simulink model "SF051A_SnsrOffsLrng"  (R2013b)
settings: Solver=FixedStepDiscrete  SolverMode=SingleTasking  StartTime=0.0  StopTime=1  FixedStep=0.002  RelTol=1e-3
values from neighbouring files (symbols this model uses):
  ARCHGLBPRM_10MILLISEC_SEC_F32 = DataDict.Constant    [SF051A_SnsrOffsLrng_DataDict.m]
  ARCHGLBPRM_2MILLISEC_SEC_F32 = DataDict.Constant    [SF051A_SnsrOffsLrng_DataDict.m]
  ARCHGLBPRM_2PI_ULS_F32 = DataDict.Constant    [SF051A_SnsrOffsLrng_DataDict.m]
  ARCHGLBPRM_FLOATZEROTHD_ULS_F32 = DataDict.Constant    [SF051A_SnsrOffsLrng_DataDict.m]
  ARCHGLBPRM_PIOVER180_ULS_F32 = DataDict.Constant    [SF051A_SnsrOffsLrng_DataDict.m]
  CNV100MICROSECTOSEC_SECPERCNT_F32 = DataDict.Constant    [SF051A_SnsrOffsLrng_DataDict.m]
  COVRAMTRXNIT_ULS_F32 = DataDict.Constant    [SF051A_SnsrOffsLrng_DataDict.m]
  HWAGHILIM_HWDEG_F32 = DataDict.Constant    [SF051A_SnsrOffsLrng_DataDict.m]
  HWAUTHYTHD_ULS_F32 = DataDict.Constant    [SF051A_SnsrOffsLrng_DataDict.m]
  HWTQLRNGSTSLRND_CNT_U08 = DataDict.Constant    [SF051A_SnsrOffsLrng_DataDict.m]
  HWTQLRNGSTSNEGOFFS_CNT_U08 = DataDict.Constant    [SF051A_SnsrOffsLrng_DataDict.m]
  HWTQLRNGSTSNOTLRND_CNT_U08 = DataDict.Constant    [SF051A_SnsrOffsLrng_DataDict.m]
  HWTQLRNGSTSPOSOFFS_CNT_U08 = DataDict.Constant    [SF051A_SnsrOffsLrng_DataDict.m]
  HWTQLRNGSTSZEROOFFS_CNT_U08 = DataDict.Constant    [SF051A_SnsrOffsLrng_DataDict.m]
  IDYMTRX_ULS_F32 = DataDict.Constant    [SF051A_SnsrOffsLrng_DataDict.m]
  IVS10MS_ULSPERSEC_F32 = DataDict.Constant    [SF051A_SnsrOffsLrng_DataDict.m]
  LRNGFILTICON_ULS_F32 = DataDict.Constant    [SF051A_SnsrOffsLrng_DataDict.m]
  ONE_ULS_F32 = DataDict.Constant    [SF051A_SnsrOffsLrng_DataDict.m]
  SnsrOffsLrnd = DataDict.NVM    [SF051A_SnsrOffsLrng_DataDict.m]
  SnsrOffsLrngFctEna = DataDict.Calibration    [SF051A_SnsrOffsLrng_DataDict.m]
  SnsrOffsLrngHwAgLrngDrvgDstThd = DataDict.Calibration    [SF051A_SnsrOffsLrng_DataDict.m]
  SnsrOffsLrngHwAgLrngEna = DataDict.Calibration    [SF051A_SnsrOffsLrng_DataDict.m]
  SnsrOffsLrngHwAgLrngHwVelThd = DataDict.Calibration    [SF051A_SnsrOffsLrng_DataDict.m]
  SnsrOffsLrngHwAgLrngSysTqThd = DataDict.Calibration    [SF051A_SnsrOffsLrng_DataDict.m]
  SnsrOffsLrngHwAgLrngSysTqThdMed = DataDict.Calibration    [SF051A_SnsrOffsLrng_DataDict.m]
  SnsrOffsLrngHwAgLrngSysTqThdTrustd = DataDict.Calibration    [SF051A_SnsrOffsLrng_DataDict.m]
  SnsrOffsLrngHwAgLrngSysTqThdWide = DataDict.Calibration    [SF051A_SnsrOffsLrng_DataDict.m]
  SnsrOffsLrngHwAgLrngTi = DataDict.Calibration    [SF051A_SnsrOffsLrng_DataDict.m]
  SnsrOffsLrngHwAgLrngVehSpdThd = DataDict.Calibration    [SF051A_SnsrOffsLrng_DataDict.m]
  SnsrOffsLrngHwAgLrngYawOffsDbnd = DataDict.Calibration    [SF051A_SnsrOffsLrng_DataDict.m]
  SnsrOffsLrngHwAgLrngYawRateThd = DataDict.Calibration    [SF051A_SnsrOffsLrng_DataDict.m]
  SnsrOffsLrngHwAgOffsLim = DataDict.Calibration    [SF051A_SnsrOffsLrng_DataDict.m]
  SnsrOffsLrngHwTqLrngEna = DataDict.Calibration    [SF051A_SnsrOffsLrng_DataDict.m]
  SnsrOffsLrngHwTqLrngEnaTiThd = DataDict.Calibration    [SF051A_SnsrOffsLrng_DataDict.m]
  SnsrOffsLrngHwTqLrngHwAgDbnd = DataDict.Calibration    [SF051A_SnsrOffsLrng_DataDict.m]
  SnsrOffsLrngHwTqLrngHwAgThd = DataDict.Calibration    [SF051A_SnsrOffsLrng_DataDict.m]
  SnsrOffsLrngHwTqLrngHwTqThd = DataDict.Calibration    [SF051A_SnsrOffsLrng_DataDict.m]
  SnsrOffsLrngHwTqLrngHwTqZeroOffsThd = DataDict.Calibration    [SF051A_SnsrOffsLrng_DataDict.m]
  SnsrOffsLrngHwTqLrngHwVelThd = DataDict.Calibration    [SF051A_SnsrOffsLrng_DataDict.m]
  SnsrOffsLrngHwTqLrngMeasTi = DataDict.Calibration    [SF051A_SnsrOffsLrng_DataDict.m]
  SnsrOffsLrngHwTqLrngMeasTiScar = DataDict.Calibration    [SF051A_SnsrOffsLrng_DataDict.m]
  SnsrOffsLrngHwTqLrngSampleImbThd1 = DataDict.Calibration    [SF051A_SnsrOffsLrng_DataDict.m]
  SnsrOffsLrngHwTqLrngSampleImbThd2 = DataDict.Calibration    [SF051A_SnsrOffsLrng_DataDict.m]
  SnsrOffsLrngHwTqLrngSampleThd1 = DataDict.Calibration    [SF051A_SnsrOffsLrng_DataDict.m]
  SnsrOffsLrngHwTqLrngSampleThd2 = DataDict.Calibration    [SF051A_SnsrOffsLrng_DataDict.m]
  SnsrOffsLrngHwTqLrngTiWghtCoeff = DataDict.Calibration    [SF051A_SnsrOffsLrng_DataDict.m]
  SnsrOffsLrngHwTqLrngVehSpdThd = DataDict.Calibration    [SF051A_SnsrOffsLrng_DataDict.m]
  SnsrOffsLrngHwTqOffsLim = DataDict.Calibration    [SF051A_SnsrOffsLrng_DataDict.m]
  SnsrOffsLrngSampleCntForHwTqLrngRst = DataDict.Calibration    [SF051A_SnsrOffsLrng_DataDict.m]
  SnsrOffsLrngTqInpDetnPwrEstimnThd = DataDict.Calibration    [SF051A_SnsrOffsLrng_DataDict.m]
  SnsrOffsLrngTqInpDetnSinGenrAmp = DataDict.Calibration    [SF051A_SnsrOffsLrng_DataDict.m]
  SnsrOffsLrngTqInpDetnSinGenrFrq = DataDict.Calibration    [SF051A_SnsrOffsLrng_DataDict.m]
  SnsrOffsLrngTqInpDetnStg1FilGain = DataDict.Calibration    [SF051A_SnsrOffsLrng_DataDict.m]
  SnsrOffsLrngTqInpDetnStg1WinSize = DataDict.Calibration    [SF051A_SnsrOffsLrng_DataDict.m]
  SnsrOffsLrngTqInpDetnStg2FilGainCen = DataDict.Calibration    [SF051A_SnsrOffsLrng_DataDict.m]
  SnsrOffsLrngTqInpDetnStg2FilGainDwn = DataDict.Calibration    [SF051A_SnsrOffsLrng_DataDict.m]
  SnsrOffsLrngTqInpDetnStg2FilGainUp = DataDict.Calibration    [SF051A_SnsrOffsLrng_DataDict.m]
  SnsrOffsLrngTqInpDetnStg2WinSize = DataDict.Calibration    [SF051A_SnsrOffsLrng_DataDict.m]
  SnsrOffsLrngYawLrngEna = DataDict.Calibration    [SF051A_SnsrOffsLrng_DataDict.m]
  SnsrOffsLrngYawLrngHwAgThd = DataDict.Calibration    [SF051A_SnsrOffsLrng_DataDict.m]
  SnsrOffsLrngYawLrngTi = DataDict.Calibration    [SF051A_SnsrOffsLrng_DataDict.m]
  SnsrOffsLrngYawLrngYawAThd = DataDict.Calibration    [SF051A_SnsrOffsLrng_DataDict.m]
  SnsrOffsLrngYawOffsFrshTiThd = DataDict.Calibration    [SF051A_SnsrOffsLrng_DataDict.m]
  SnsrOffsLrngYawRateOffsLim = DataDict.Calibration    [SF051A_SnsrOffsLrng_DataDict.m]
  SPDCNVN_MTRPERSECPERKPH_F32 = DataDict.Constant    [SF051A_SnsrOffsLrng_DataDict.m]
  SysGlbPrmSysTqRat = DataDict.ImprtdCal    [SF051A_SnsrOffsLrng_DataDict.m]
  TISTEP10MS_MINS_F32 = DataDict.Constant    [SF051A_SnsrOffsLrng_DataDict.m]
  TQINPDETNLOGGAIN_ULS_F32 = DataDict.Constant    [SF051A_SnsrOffsLrng_DataDict.m]
  YAWELPDTIHILIM_MINS_F32 = DataDict.Constant    [SF051A_SnsrOffsLrng_DataDict.m]
  YAWRATENOISE_VEHDEGPERSEC_F32 = DataDict.Constant    [SF051A_SnsrOffsLrng_DataDict.m]
  ZERO_ULS_F32 = DataDict.Constant    [SF051A_SnsrOffsLrng_DataDict.m]
  ZEROVECT_ULS_F32 = DataDict.Constant    [SF051A_SnsrOffsLrng_DataDict.m]
undefined symbols (not defined in the file or in its folder): NvmGetErrSts1
libraries: Fil x34, NxtrLim x20, FixdToFloat x17, FloatToFixd x16, simulink x12, NxtrAbslt x12, NxtrNvM x8, NxtrMath x3
(part 7 of 12)

== system SF051A_SnsrOffsLrng/SnsrOffsLrng/SnsrOffsLrngPer2/Enable_Function/YOC ==
  note: Every execution loop of Periodic 2, the yaw rate freshness timer increments.  Using a loop counter instead of client calls
      | because the elapsed time is "frozen" across ignition cycles.  The counter is reset to zero when learning occurs.
  note: When vehicle conditions are right and all bus signals are valid, begin or continue learning.
  YawRateLrngEna : Inport
  YawRateFild : Inport  RequirementInfo="{'linktype_rmi_doors' '0000babd (/E-STEER Core/SubSystem Specifications/Application Functions/SF051A Sensor Offset Learning)' '#SF051A_100' 'true' 'REQ:  SF051A_100' '' } %GIDa_4788fb8c_6bdd_419e_be01_c723b642e277"  Port=2
  YawA : Inport  RequirementInfo="{'linktype_rmi_doors' '0000babd (/E-STEER Core/SubSystem Specifications/Application Functions/SF051A Sensor Offset Learning)' '#SF051A_99' 'true' 'REQ:  SF051A_99' '' } %GIDa_1132fb7b_54bf_40b1_acf5_f9054bb6ad26"  Port=3
  VehSpd : Inport  RequirementInfo="{'linktype_rmi_doors' '0000babd (/E-STEER Core/SubSystem Specifications/Application Functions/SF051A Sensor Offset Learning)' '#SF051A_102' 'true' 'REQ:  SF051A_102' '' } %GIDa_5315707f_4311_4e1a_9598_78d874dd3bdb"  Port=4
  HwAg : Inport  RequirementInfo="{'linktype_rmi_doors' '0000babd (/E-STEER Core/SubSystem Specifications/Application Functions/SF051A Sensor Offset Learning)' '#SF051A_101' 'true' 'REQ:  SF051A_101' '' } %GIDa_72eb9de4_dd58_44cc_88ca_111522a15ca4"  Port=5
  Add : Sum
  Constant : Constant  RequirementInfo="{'linktype_rmi_doors' '0000babd (/E-STEER Core/SubSystem Specifications/Application Functions/SF051A Sensor Offset Learning)' '#SF051A_111' 'true' 'REQ:  SF051A_111' '' ; 'linktype_rmi_doors' '0000babd (/E-STEER Core/SubSystem Specifications/Application Functions/SF051A Sensor Offset Learning)' '#SF051A_242' 'true' 'REQ:  SF051A_242' '' } %GIDa_883fb207_2bdb_43f4_8fbf_3d3c8800e308"  Value=SnsrOffsLrngYawOffsFrshTiThd  OutDataTypeStr=single
  Constant1 : Constant  Value=TISTEP10MS_MINS_F32  OutDataTypeStr=single
  Data Store Read : DataStoreRead  DataStoreName=SnsrOffsLrnd  DataStoreElements=SnsrOffsLrnd.YawRateElpdTi
  Data Store Write : DataStoreWrite  DataStoreName=SnsrOffsLrnd  DataStoreElements=SnsrOffsLrnd.YawRateElpdTi
  Data Store Write1 : DataStoreWrite  RequirementInfo="{'linktype_rmi_doors' '0000babd (/E-STEER Core/SubSystem Specifications/Application Functions/SF051A Sensor Offset Learning)' '#SF051A_112' 'true' 'REQ:  SF051A_112' '' } %GIDa_1386d18f_d052_4548_b025_86f8f1b54bd3"  DataStoreName=VehYawRateOffsFrsh
  Do nothing : Subsystem  TreatAsAtomicUnit=on
  If : If  RequirementInfo="{'linktype_rmi_doors' '0000babd (/E-STEER Core/SubSystem Specifications/Application Functions/SF051A Sensor Offset Learning)' '#SF051A_95' 'true' 'REQ:  SF051A_95' '' } %GIDa_5a0d1c96_ac6c_4e69_b879_396e00cbc286"  NumInputs=2  IfExpression=u1 & u2
  Learn : Subsystem  RequirementInfo="{'linktype_rmi_doors' '0000babd (/E-STEER Core/SubSystem Specifications/Application Functions/SF051A Sensor Offset Learning)' '#SF051A_94' 'true' 'REQ:  SF051A_94' '' } %GIDa_548ddfb5_a741_4714_aec1_02ee3ee42dbb"  TreatAsAtomicUnit=on
  Learning Conditions : Subsystem  RequirementInfo="{'linktype_rmi_doors' '0000babd (/E-STEER Core/SubSystem Specifications/Application Functions/SF051A Sensor Offset Learning)' '#SF051A_97' 'true' 'REQ:  SF051A_97' '' ; 'linktype_rmi_doors' '0000babd (/E-STEER Core/SubSystem Specifications/Application Functions/SF051A Sensor Offset Learning)' '#SF051A_96' 'true' 'REQ:  SF051A_96' '' } %GIDa_890fa9a9_e67d_4d09_8fef_362b51c9d8ff"
  LimStat_f32 : NxtrLim/LimStat_f32  LoLim=ZERO_ULS_F32  HiLim=SnsrOffsLrngYawOffsFrshTiThd
      settings: AttributesFormatString=|
      | Low Limit: %<LoLim>
      | High Limit:%<HiLim>
  Relational Operator : RelationalOperator  RequirementInfo="{'linktype_rmi_doors' '0000babd (/E-STEER Core/SubSystem Specifications/Application Functions/SF051A Sensor Offset Learning)' '#SF051A_111' 'true' 'REQ:  SF051A_111' '' ; 'linktype_rmi_doors' '0000babd (/E-STEER Core/SubSystem Specifications/Application Functions/SF051A Sensor Offset Learning)' '#SF051A_242' 'true' 'REQ:  SF051A_242' '' } %GIDa_100189d6_4f90_49af_8752_2852919b8786"  Operator=<=  OutDataTypeStr=boolean
  Subsystem5 : Subsystem  Description=|  mask(Copyright Information){none=on}
      | Copyright info block.                                               
      |                                                                     
      | Place copyright information at the top of every subsystem in design.
      mask prompts: none "No parameters"
      mask help: Place copyright information at the top of every subsystem in design.
      mask Display:
      | NxtrConf = 'Nexteer Confidential';
      | 
      | sys = bdroot; %handle for the current model ("system")
      | first = get_param(sys,'Created');
      | first = first(end-3:end);  %year is last four digits
      | 
      | last = get_param(sys,'LastModifiedDate');
      | if isempty(last)
      |     last = datestr(now,'yyyy');
      | else
      |     last = last(end-3:end);
      | end
      | 
      | if strcmp(first,last)
      |     fprintf('%s -- Copyright %s Nexteer',NxtrConf,first)
      | else
      |     fprintf('%s -- %s%s- %s Nexteer',NxtrConf,char(169),first,last)
      | end
  wires:
  YawRateFild/1 -> Learning Conditions/4(YawRateFild), Learn/1(YawRate)
  Learning Conditions/1(LrngCdnVld) -> If/2
  YawRateLrngEna/1 -> If/1
  VehSpd/1 -> Learning Conditions/1(VehSpd)
  HwAg/1 -> Learning Conditions/2(HwAg)
  If/1 -> Learn/Action
  Constant/1 -> Relational Operator/2
  Data Store Read/1 -> Add/1
  Constant1/1 -> Add/2
  Add/1 -> LimStat_f32/1, Relational Operator/1  "ElpsdTi"
  LimStat_f32/1 -> Data Store Write/1
  YawA/1 -> Learning Conditions/3(YawA)
  If/2 -> Do nothing/Action
  Relational Operator/1 -> Data Store Write1/1

== system SF051A_SnsrOffsLrng/SnsrOffsLrng/SetHwTqOffs/Reset Learning/GetRefTmr100MicroSec32bit/CopyRight2 ==

== system SF051A_SnsrOffsLrng/SnsrOffsLrng/SnsrOffsLrngInit1/NVM Management/Data Invalid/Subsystem5 ==

== system SF051A_SnsrOffsLrng/SnsrOffsLrng/SnsrOffsLrngInit1/NVM Management/Data Valid/Subsystem5 ==

== system SF051A_SnsrOffsLrng/SnsrOffsLrng/SnsrOffsLrngInit1/NVM Management/Not Enabled/Subsystem5 ==

== system SF051A_SnsrOffsLrng/SnsrOffsLrng/SnsrOffsLrngPer1/EnableLearning/Default_TqInpDetn/Subsystem5 ==

== system SF051A_SnsrOffsLrng/SnsrOffsLrng/SnsrOffsLrngPer1/EnableLearning/EnablingConditions/CheckLastMeasHwPos ==
  HwAg : Inport
  Abslt_f32_f32 : NxtrAbslt/Abslt_f32_f32  SFunctionSpec=single y1 = Abslt_f32_f32(single u1)
      settings: AttributesFormatString=%<Name>
  Constant : Constant  Value=SnsrOffsLrngHwTqLrngHwAgDbnd
  Data Store Read : DataStoreRead  DataStoreName=SnsrOffsLrnd  DataStoreElements=SnsrOffsLrnd.HwTqLrngHwAgRef
  FalseOut_KeepRef : Subsystem  TreatAsAtomicUnit=on
  FixdToFloat_f32_s16 : FixdToFloat/FixdToFloat_f32_s16  Param1=4
  If : If  IfExpression=u1
  Merge : Merge
  Relational Operator : RelationalOperator  OutDataTypeStr=boolean
  Subsystem5 : Subsystem  Description=|  mask(Copyright Information){none=on}
      | Copyright info block.                                               
      |                                                                     
      | Place copyright information at the top of every subsystem in design.
      mask prompts: none "No parameters"
      mask help: Place copyright information at the top of every subsystem in design.
      mask Display:
      | NxtrConf = 'Nexteer Confidential';
      | 
      | sys = bdroot; %handle for the current model ("system")
      | first = get_param(sys,'Created');
      | first = first(end-3:end);  %year is last four digits
      | 
      | last = get_param(sys,'LastModifiedDate');
      | if isempty(last)
      |     last = datestr(now,'yyyy');
      | else
      |     last = last(end-3:end);
      | end
      | 
      | if strcmp(first,last)
      |     fprintf('%s -- Copyright %s Nexteer',NxtrConf,first)
      | else
      |     fprintf('%s -- %s%s- %s Nexteer',NxtrConf,char(169),first,last)
      | end
  Subtract : Sum  Inputs=+-
  TrueOut_ResetRef : Subsystem  TreatAsAtomicUnit=on
  HwAgMoved : Outport
  wires:
  Relational Operator/1 -> If/1
  Constant/1 -> Relational Operator/2
  Data Store Read/1 -> FixdToFloat_f32_s16/1
  HwAg/1 -> Subtract/1
  Subtract/1 -> Abslt_f32_f32/1
  Abslt_f32_f32/1 -> Relational Operator/1
  If/1 -> TrueOut_ResetRef/Action
  TrueOut_ResetRef/1(HwAgMoved) -> Merge/1
  FalseOut_KeepRef/1(HwAgMoved) -> Merge/2
  If/2 -> FalseOut_KeepRef/Action
  Merge/1 -> HwAgMoved/1
  FixdToFloat_f32_s16/1 -> Subtract/2

== system SF051A_SnsrOffsLrng/SnsrOffsLrng/SnsrOffsLrngPer1/EnableLearning/EnablingConditions/Subsystem5 ==

== system SF051A_SnsrOffsLrng/SnsrOffsLrng/SnsrOffsLrngPer1/EnableLearning/Eval_Time/GetTiSpan100MicroSec32bit ==
  note: Subtract original reference time
  note: seconds
  note: microseconds
  note: counts
  note: Wrap-to-zero
  note: 1 count = 100 uSec
  note: Get current system time
  note: GetTiSpan100MicroSec32bit
  note: Created Aug 18, 2015
      | Modified Oct 21, 2015
      | Modified Oct 30, 2015
      | Kevin Derry
  RefTmr : Inport
  CopyRight2 : Subsystem  Description=|  mask(Copyright Information){none=on}
      | Copyright info block.                                               
      |                                                                     
      | Place copyright information at the top of every subsystem in design.
      mask prompts: none "No parameters"
      mask help: Place copyright information at the top of every subsystem in design.
      mask Display:
      | NxtrConf = 'Nexteer Confidential';
      | 
      | sys = bdroot; %handle for the current model ("system")
      | first = get_param(sys,'Created');
      | if(isempty(first))
      |     first = datestr(now,'yyyy');
      | else
      |     first = first(end-3:end);  %year is last four digits
      | end
      | 
      | last = get_param(sys,'LastModifiedDate');
      | if isempty(last)
      |     last = datestr(now,'yyyy');
      | else
      |     last = last(end-3:end);
      | end
      | 
      | if strcmp(first,last)
      |     fprintf('%s -- Copyright %s Nexteer',NxtrConf,first)
      | else
      |     fprintf('%s -- %s%s- %s Nexteer',NxtrConf,char(169),first,last)
      | end
  Count per uSec : Constant  Value=0.01
  Data Store Read1 : DataStoreRead  DataStoreName=SimnTi
  Data Type Conversion2 : DataTypeConversion  OutDataTypeStr=uint32
  Divide1 : Product  Inputs=**
  Divide2 : Product  Inputs=*/
  If : If  NumInputs=2  IfExpression=u1 >= u2
  Max Counts : Constant  Value=2^32-1
  Merge : Merge
  No wrapping : Subsystem  TreatAsAtomicUnit=on
  Product2 : Product
  Product3 : Product
  Rounding : Rounding
  Subtract3 : Sum  Inputs=+-
  Wrapping : Subsystem  TreatAsAtomicUnit=on
  uSec per Sec : Constant  Value=1000000
  TiSpan : Outport
  wires:
  Wrapping/1(Out1) -> Merge/2
  No wrapping/1(Out1) -> Merge/1
  If/2 -> Wrapping/Action
  If/1 -> No wrapping/Action
  Product3/1 -> Subtract3/2
  Subtract3/1 -> Data Type Conversion2/1
  Rounding/1 -> Product3/1
  Divide2/1 -> Rounding/1
  Max Counts/1 -> Divide2/2, Product3/2
  Divide1/1 -> Divide2/1, Subtract3/1
  Product2/1 -> Divide1/1
  Data Store Read1/1 -> Product2/1
  Count per uSec/1 -> Divide1/2
  uSec per Sec/1 -> Product2/2
  Merge/1 -> TiSpan/1
  RefTmr/1 -> If/2, No wrapping/2(ref), Wrapping/2(ref)
  Data Type Conversion2/1 -> If/1, No wrapping/1(new), Wrapping/1(new)

== system SF051A_SnsrOffsLrng/SnsrOffsLrng/SnsrOffsLrngPer1/EnableLearning/Eval_Time/Subsystem5 ==

== system SF051A_SnsrOffsLrng/SnsrOffsLrng/SnsrOffsLrngPer1/EnableLearning/False_Reset/GetRefTmr100MicroSec32bit ==
  note: 1 count = 100 uSec
  note: seconds
  note: microseconds
  note: counts
  note: Wrap-to-zero
  note: GetRefTmr100MicroSec32bit
  note: Created Aug 18, 2015
      | Modified Oct 21, 2015
      | Modified Oct 30, 2015
      | Kevin Derry
  CopyRight2 : Subsystem  Description=|  mask(Copyright Information){none=on}
      | Copyright info block.                                               
      |                                                                     
      | Place copyright information at the top of every subsystem in design.
      mask prompts: none "No parameters"
      mask help: Place copyright information at the top of every subsystem in design.
      mask Display:
      | NxtrConf = 'Nexteer Confidential';
      | 
      | sys = bdroot; %handle for the current model ("system")
      | first = get_param(sys,'Created');
      | if(isempty(first))
      |     first = datestr(now,'yyyy');
      | else
      |     first = first(end-3:end);  %year is last four digits
      | end
      | 
      | last = get_param(sys,'LastModifiedDate');
      | if isempty(last)
      |     last = datestr(now,'yyyy');
      | else
      |     last = last(end-3:end);
      | end
      | 
      | if strcmp(first,last)
      |     fprintf('%s -- Copyright %s Nexteer',NxtrConf,first)
      | else
      |     fprintf('%s -- %s%s- %s Nexteer',NxtrConf,char(169),first,last)
      | end
  Count per uSec : Constant  Value=0.01
  Data Store Read1 : DataStoreRead  DataStoreName=SimnTi
  Data Type Conversion1 : DataTypeConversion  OutDataTypeStr=uint32
  Divide1 : Product  Inputs=**
  Divide2 : Product  Inputs=*/
  Max Counts : Constant  Value=2^32-1
  Product1 : Product
  Product2 : Product
  Rounding : Rounding
  Subtract1 : Sum  Inputs=+-
  uSec per Sec : Constant  Value=1000000
  RefTmr : Outport
  wires:
  Product2/1 -> Subtract1/2
  Subtract1/1 -> Data Type Conversion1/1
  Rounding/1 -> Product2/1
  Divide2/1 -> Rounding/1
  Max Counts/1 -> Divide2/2, Product2/2
  Divide1/1 -> Divide2/1, Subtract1/1
  Product1/1 -> Divide1/1
  Count per uSec/1 -> Divide1/2
  uSec per Sec/1 -> Product1/2
  Data Type Conversion1/1 -> RefTmr/1
  Data Store Read1/1 -> Product1/1

== system SF051A_SnsrOffsLrng/SnsrOffsLrng/SnsrOffsLrngPer1/EnableLearning/False_Reset/Subsystem5 ==

== system SF051A_SnsrOffsLrng/SnsrOffsLrng/SnsrOffsLrngPer1/EnableLearning/Filter_HwTq/Subsystem5 ==

== system SF051A_SnsrOffsLrng/SnsrOffsLrng/SnsrOffsLrngPer1/EnableLearning/Perform_TqInpDetn/Do nothing ==
  Action Port : ActionPort  ActionType=else
  Subsystem5 : Subsystem  Description=|  mask(Copyright Information){none=on}
      | Copyright info block.                                               
      |                                                                     
      | Place copyright information at the top of every subsystem in design.
      mask prompts: none "No parameters"
      mask help: Place copyright information at the top of every subsystem in design.
      mask Display:
      | NxtrConf = 'Nexteer Confidential';
      | 
      | sys = bdroot; %handle for the current model ("system")
      | first = get_param(sys,'Created');
      | first = first(end-3:end);  %year is last four digits
      | 
      | last = get_param(sys,'LastModifiedDate');
      | if isempty(last)
      |     last = datestr(now,'yyyy');
      | else
      |     last = last(end-3:end);
      | end
      | 
      | if strcmp(first,last)
      |     fprintf('%s -- Copyright %s Nexteer',NxtrConf,first)
      | else
      |     fprintf('%s -- %s%s- %s Nexteer',NxtrConf,char(169),first,last)
      | end

== system SF051A_SnsrOffsLrng/SnsrOffsLrng/SnsrOffsLrngPer1/EnableLearning/Perform_TqInpDetn/ElapsedTime ==
  Add : Sum
  Data Store Read : DataStoreRead  DataStoreName=TqInpDetnEnaTi
  Data Store Write : DataStoreWrite  DataStoreName=TqInpDetnEnaTi
  LimStat_f32 : NxtrLim/LimStat_f32  LoLim=ZERO_ULS_F32  HiLim=HWTQLRNGTMRHILIM_SEC_F32
      settings: AttributesFormatString=|
      | Low Limit: %<LoLim>
      | High Limit:%<HiLim>
  Subsystem5 : Subsystem  Description=|  mask(Copyright Information){none=on}
      | Copyright info block.                                               
      |                                                                     
      | Place copyright information at the top of every subsystem in design.
      mask prompts: none "No parameters"
      mask help: Place copyright information at the top of every subsystem in design.
      mask Display:
      | NxtrConf = 'Nexteer Confidential';
      | 
      | sys = bdroot; %handle for the current model ("system")
      | first = get_param(sys,'Created');
      | first = first(end-3:end);  %year is last four digits
      | 
      | last = get_param(sys,'LastModifiedDate');
      | if isempty(last)
      |     last = datestr(now,'yyyy');
      | else
      |     last = last(end-3:end);
      | end
      | 
      | if strcmp(first,last)
      |     fprintf('%s -- Copyright %s Nexteer',NxtrConf,first)
      | else
      |     fprintf('%s -- %s%s- %s Nexteer',NxtrConf,char(169),first,last)
      | end
  Ts : Constant  Value=ARCHGLBPRM_2MILLISEC_SEC_F32
  TiEnad : Outport
  wires:
  Ts/1 -> Add/1
  Data Store Read/1 -> Add/2
  Add/1 -> LimStat_f32/1
  LimStat_f32/1 -> TiEnad/1, Data Store Write/1

== system SF051A_SnsrOffsLrng/SnsrOffsLrng/SnsrOffsLrngPer1/EnableLearning/Perform_TqInpDetn/Enable_PreProcessing ==
  note: Enable_PreProcessing == true
  TiEnad : Inport
  HwTqFild : Inport  Port=2
  Constant : Constant  Value=SnsrOffsLrngTqInpDetnPwrEstimnThd
  Constant2 : Constant  Value=ARCHGLBPRM_2MILLISEC_SEC_F32
  Display : DataStoreWrite  DataStoreName=dSnsrOffsLrngTqInpPrsntRaw
  False_Hold : Subsystem  TreatAsAtomicUnit=on
  If : If  NumInputs=2  IfExpression=u1 & u2  ElseIfExpressions=u1 & ~u2
  Merge_Present : Merge  Inputs=3
  Merge_Validity : Merge  Inputs=3
  Preprocessing : Subsystem
  Product : Product
  Relational Operator : RelationalOperator  OutDataTypeStr=boolean
  Relational Operator1 : RelationalOperator  Operator=>  OutDataTypeStr=boolean
  Subsystem5 : Subsystem  Description=|  mask(Copyright Information){none=on}
      | Copyright info block.                                               
      |                                                                     
      | Place copyright information at the top of every subsystem in design.
      mask prompts: none "No parameters"
      mask help: Place copyright information at the top of every subsystem in design.
      mask Display:
      | NxtrConf = 'Nexteer Confidential';
      | 
      | sys = bdroot; %handle for the current model ("system")
      | first = get_param(sys,'Created');
      | first = first(end-3:end);  %year is last four digits
      | 
      | last = get_param(sys,'LastModifiedDate');
      | if isempty(last)
      |     last = datestr(now,'yyyy');
      | else
      |     last = last(end-3:end);
      | end
      | 
      | if strcmp(first,last)
      |     fprintf('%s -- Copyright %s Nexteer',NxtrConf,first)
      | else
      |     fprintf('%s -- %s%s- %s Nexteer',NxtrConf,char(169),first,last)
      | end
  True_False : Subsystem  TreatAsAtomicUnit=on
  True_True : Subsystem  TreatAsAtomicUnit=on
  TqInpPrsntVld : Outport  InitialOutput=0
  TqInpPrsnt : Outport  Port=2  InitialOutput=0
  wires:
  Preprocessing/2(HwTrqPreproc) -> Relational Operator1/1
  HwTqFild/1 -> Preprocessing/1(HwTqFild)
  Product/1 -> Relational Operator/2  "TqInpDetnBufTi"
  TiEnad/1 -> Relational Operator/1
  If/3 -> False_Hold/Action
  If/1 -> True_True/Action
  Relational Operator/1 -> If/1  "HwTqPreprocVld"
  Constant/1 -> Relational Operator1/2
  Relational Operator1/1 -> If/2, Display/1  "TqInpPrsntRaw"
  If/2 -> True_False/Action
  True_True/1(Vld) -> Merge_Validity/1
  True_False/1(Vld) -> Merge_Validity/2
  False_Hold/1(Vld) -> Merge_Validity/3
  Merge_Validity/1 -> TqInpPrsntVld/1
  True_True/2(Prsnt) -> Merge_Present/1
  True_False/2(Prsnt) -> Merge_Present/2
  False_Hold/2(Prsnt) -> Merge_Present/3
  Merge_Present/1 -> TqInpPrsnt/1
  Preprocessing/1(SampleCntrLim) -> Product/2
  Constant2/1 -> Product/1

== system SF051A_SnsrOffsLrng/SnsrOffsLrng/SnsrOffsLrngPer1/EnableLearning/Perform_TqInpDetn/SetStuffToZero ==
  Action Port : ActionPort  ActionType=then
  Constant : Constant  Value=ZERO_ULS_F32  OutDataTypeStr=single
      settings: AttributesFormatString=%<OutDataTypeStr>
  Constant1 : Constant  Value=0  OutDataTypeStr=uint16
      settings: AttributesFormatString=%<OutDataTypeStr>
  Constant2 : Constant  Value=0*(1:72)  OutDataTypeStr=single
      settings: AttributesFormatString=%<OutDataTypeStr>
  Constant3 : Constant  Value=true  OutDataTypeStr=boolean
      settings: AttributesFormatString=%<OutDataTypeStr>
  Constant4 : Constant  Value=0  OutDataTypeStr=uint8
      settings: AttributesFormatString=%<OutDataTypeStr>
  Data Store Write : DataStoreWrite  DataStoreName=TqInpDetnEnaTi
  Data Store Write1 : DataStoreWrite  DataStoreName=TqInpDetnHwTqFil  DataStoreElements=TqInpDetnHwTqFil.FilSt
  Data Store Write10 : DataStoreWrite  DataStoreName=TqInpDetnStg2UpFilSt2
  Data Store Write11 : DataStoreWrite  DataStoreName=TqInpDetnStg2UpFilSt1
  Data Store Write12 : DataStoreWrite  DataStoreName=TqInpDetnStg2CenFilSt1
  Data Store Write13 : DataStoreWrite  DataStoreName=TqInpDetnHwTqPreProc
  Data Store Write14 : DataStoreWrite  DataStoreName=TqInpDetnStg2DwnFilSt1
  Data Store Write15 : DataStoreWrite  DataStoreName=TqInpDetnStg2CenFilSt2
  Data Store Write2 : DataStoreWrite  DataStoreName=TqInpDetnPreProcEnaLoop
  Data Store Write4 : DataStoreWrite  DataStoreName=TqInpDetnSinGenrAg
  Data Store Write5 : DataStoreWrite  DataStoreName=TqInpDetnStg1Buf
  Data Store Write6 : DataStoreWrite  DataStoreName=TqInpDetnStg1Idx
  Data Store Write7 : DataStoreWrite  DataStoreName=TqInpDetnStg1FilSt2
  Data Store Write8 : DataStoreWrite  DataStoreName=TqInpDetnStg1FilSt1
  Data Store Write9 : DataStoreWrite  DataStoreName=TqInpDetnStg2DwnFilSt2
  StateVariable : DataStoreWrite  DataStoreName=HwTqLrngTqInpPrsnt
  Subsystem5 : Subsystem  Description=|  mask(Copyright Information){none=on}
      | Copyright info block.                                               
      |                                                                     
      | Place copyright information at the top of every subsystem in design.
      mask prompts: none "No parameters"
      mask help: Place copyright information at the top of every subsystem in design.
      mask Display:
      | NxtrConf = 'Nexteer Confidential';
      | 
      | sys = bdroot; %handle for the current model ("system")
      | first = get_param(sys,'Created');
      | first = first(end-3:end);  %year is last four digits
      | 
      | last = get_param(sys,'LastModifiedDate');
      | if isempty(last)
      |     last = datestr(now,'yyyy');
      | else
      |     last = last(end-3:end);
      | end
      | 
      | if strcmp(first,last)
      |     fprintf('%s -- Copyright %s Nexteer',NxtrConf,first)
      | else
      |     fprintf('%s -- %s%s- %s Nexteer',NxtrConf,char(169),first,last)
      | end
  wires:
  Constant1/1 -> Data Store Write2/1
  Constant/1 -> Data Store Write1/1, Data Store Write13/1, Data Store Write11/1, Data Store Write10/1, Data Store Write12/1, Data Store Write15/1, Data Store Write14/1, Data Store Write9/1, Data Store Write8/1, Data Store Write7/1, Data Store Write4/1, Data Store Write/1
  Constant2/1 -> Data Store Write5/1
  Constant3/1 -> StateVariable/1
  Constant4/1 -> Data Store Write6/1

== system SF051A_SnsrOffsLrng/SnsrOffsLrng/SnsrOffsLrngPer1/EnableLearning/Perform_TqInpDetn/Subsystem5 ==

== system SF051A_SnsrOffsLrng/SnsrOffsLrng/SnsrOffsLrngPer1/Learning/CalculateOnCenterTorqueDrift/Subsystem5 ==

== system SF051A_SnsrOffsLrng/SnsrOffsLrng/SnsrOffsLrngPer1/Learning/Counter/Increment_SampleCntNeg ==
  Action Port : ActionPort  ActionType=else
  " Constant" : Constant  OutDataTypeStr=uint16
      settings: AttributesFormatString=%<OutDataTypeStr>
  Add : Sum
  Data Store Read : DataStoreRead  DataStoreName=SnsrOffsLrnd  DataStoreElements=SnsrOffsLrnd.HwTqLrngSampleCntNeg
  Data Store Write : DataStoreWrite  DataStoreName=SnsrOffsLrnd  DataStoreElements=SnsrOffsLrnd.HwTqLrngSampleCntNeg
  Subsystem5 : Subsystem  Description=|  mask(Copyright Information){none=on}
      | Copyright info block.                                               
      |                                                                     
      | Place copyright information at the top of every subsystem in design.
      mask prompts: none "No parameters"
      mask help: Place copyright information at the top of every subsystem in design.
      mask Display:
      | NxtrConf = 'Nexteer Confidential';
      | 
      | sys = bdroot; %handle for the current model ("system")
      | first = get_param(sys,'Created');
      | first = first(end-3:end);  %year is last four digits
      | 
      | last = get_param(sys,'LastModifiedDate');
      | if isempty(last)
      |     last = datestr(now,'yyyy');
      | else
      |     last = last(end-3:end);
      | end
      | 
      | if strcmp(first,last)
      |     fprintf('%s -- Copyright %s Nexteer',NxtrConf,first)
      | else
      |     fprintf('%s -- %s%s- %s Nexteer',NxtrConf,char(169),first,last)
      | end
  Size : Outport
  wires:
  " Constant"/1 -> Add/1
  Add/1 -> Size/1, Data Store Write/1
  Data Store Read/1 -> Add/2

== system SF051A_SnsrOffsLrng/SnsrOffsLrng/SnsrOffsLrngPer1/Learning/Counter/Increment_SampleCntPos ==
  Action Port : ActionPort  ActionType=then
  "  Constant" : Constant  OutDataTypeStr=uint16
      settings: AttributesFormatString=%<OutDataTypeStr>
  Add : Sum
  Data Store Read : DataStoreRead  DataStoreName=SnsrOffsLrnd  DataStoreElements=SnsrOffsLrnd.HwTqLrngSampleCntPos
  Data Store Write : DataStoreWrite  DataStoreName=SnsrOffsLrnd  DataStoreElements=SnsrOffsLrnd.HwTqLrngSampleCntPos
  Subsystem5 : Subsystem  Description=|  mask(Copyright Information){none=on}
      | Copyright info block.                                               
      |                                                                     
      | Place copyright information at the top of every subsystem in design.
      mask prompts: none "No parameters"
      mask help: Place copyright information at the top of every subsystem in design.
      mask Display:
      | NxtrConf = 'Nexteer Confidential';
      | 
      | sys = bdroot; %handle for the current model ("system")
      | first = get_param(sys,'Created');
      | first = first(end-3:end);  %year is last four digits
      | 
      | last = get_param(sys,'LastModifiedDate');
      | if isempty(last)
      |     last = datestr(now,'yyyy');
      | else
      |     last = last(end-3:end);
      | end
      | 
      | if strcmp(first,last)
      |     fprintf('%s -- Copyright %s Nexteer',NxtrConf,first)
      | else
      |     fprintf('%s -- %s%s- %s Nexteer',NxtrConf,char(169),first,last)
      | end
  Size : Outport
  wires:
  "  Constant"/1 -> Add/1
  Add/1 -> Data Store Write/1, Size/1
  Data Store Read/1 -> Add/2

== system SF051A_SnsrOffsLrng/SnsrOffsLrng/SnsrOffsLrngPer1/Learning/Counter/Subsystem5 ==

== system SF051A_SnsrOffsLrng/SnsrOffsLrng/SnsrOffsLrngPer1/Learning/Do nothing/Subsystem5 ==

== system SF051A_SnsrOffsLrng/SnsrOffsLrng/SnsrOffsLrngPer1/Learning/ForgettingFactor/ResetHwTqLrng ==
  note: LPFs
  note: State Variables
  note: NVM
  Action Port : ActionPort  ActionType=then
  Constant1 : Constant  Value=ZERO_ULS_F32  OutDataTypeStr=single
      settings: AttributesFormatString=%<OutDataTypeStr>
  Constant10 : Constant  Value=true  OutDataTypeStr=boolean
      settings: AttributesFormatString=%<OutDataTypeStr>
  Constant3 : Constant  Value=HWAGHILIM_HWDEG_F32  OutDataTypeStr=single
      settings: AttributesFormatString=%<OutDataTypeStr>
  Constant4 : Constant  Value=IDYMTRX_ULS_F32  VectorParams1D=off  OutDataTypeStr=single
      settings: AttributesFormatString=%<OutDataTypeStr>, 3x3
  Constant5 : Constant  Value=0  OutDataTypeStr=uint16
      settings: AttributesFormatString=%<OutDataTypeStr>
  Constant7 : Constant  Value=ZEROVECT_ULS_F32  VectorParams1D=off  OutDataTypeStr=single
      settings: AttributesFormatString=%<OutDataTypeStr>, 3x1
  Constant8 : Constant  Value=COVRAMTRXNIT_ULS_F32  OutDataTypeStr=single
      settings: AttributesFormatString=%<OutDataTypeStr>
  Constant9 : Constant  Value=false  OutDataTypeStr=boolean
      settings: AttributesFormatString=%<OutDataTypeStr>
  Data Store Write1 : DataStoreWrite  DataStoreName=HwTqLrngEnaTmrRef
  Data Store Write10 : DataStoreWrite  DataStoreName=HwTqLrngTqInpPrsnt
  Data Store Write2 : DataStoreWrite  DataStoreName=HwTqLrngMeasTmrRef
  Data Store Write4 : DataStoreWrite  DataStoreName=HwAgMeasFil1  DataStoreElements=HwAgMeasFil1.FilSt
  Data Store Write5 : DataStoreWrite  DataStoreName=HwAgMeasFil2  DataStoreElements=HwAgMeasFil2.FilSt
  Data Store Write6 : DataStoreWrite  DataStoreName=HwTqMeasFil1  DataStoreElements=HwTqMeasFil1.FilSt
  Data Store Write7 : DataStoreWrite  DataStoreName=HwTqMeasFil2  DataStoreElements=HwTqMeasFil2.FilSt
  Data Store Write8 : DataStoreWrite  DataStoreName=HwTqLrngTqInpDetnEnaPrev
  Data Store Write9 : DataStoreWrite  DataStoreName=TqInpDetnHwTqFil  DataStoreElements=TqInpDetnHwTqFil.FilSt
  FloatToFixd_s16_f32 : FloatToFixd/FloatToFixd_s16_f32  Param1=4
  GetRefTmr100MicroSec32bit : Subsystem
  Product : Product
  Subsystem5 : Subsystem  Description=|  mask(Copyright Information){none=on}
      | Copyright info block.                                               
      |                                                                     
      | Place copyright information at the top of every subsystem in design.
      mask prompts: none "No parameters"
      mask help: Place copyright information at the top of every subsystem in design.
      mask Display:
      | NxtrConf = 'Nexteer Confidential';
      | 
      | sys = bdroot; %handle for the current model ("system")
      | first = get_param(sys,'Created');
      | first = first(end-3:end);  %year is last four digits
      | 
      | last = get_param(sys,'LastModifiedDate');
      | if isempty(last)
      |     last = datestr(now,'yyyy');
      | else
      |     last = last(end-3:end);
      | end
      | 
      | if strcmp(first,last)
      |     fprintf('%s -- Copyright %s Nexteer',NxtrConf,first)
      | else
      |     fprintf('%s -- %s%s- %s Nexteer',NxtrConf,char(169),first,last)
      | end
  Update NVM RAM : DataStoreWrite  DataStoreName=SnsrOffsLrnd  DataStoreElements=SnsrOffsLrnd.HwTqLrngSampleCntNeg#SnsrOffsLrnd.HwTqLrngSampleCntPos#SnsrOffsLrnd.HwTqLrngHwAgRef#SnsrOffsLrnd.HwTqLrngEstimnVect(:,:)#SnsrOffsLrnd.HwTqLrngCovariMtrx(:,:)
  wires:
  Constant1/1 -> Data Store Write9/1, Data Store Write7/1, Data Store Write6/1, Data Store Write5/1, Data Store Write4/1
  GetRefTmr100MicroSec32bit/1(RefTmr) -> Data Store Write2/1, Data Store Write1/1
  Constant3/1 -> FloatToFixd_s16_f32/1
  Constant5/1 -> Update NVM RAM/1, Update NVM RAM/2
  Constant4/1 -> Product/1
  Constant8/1 -> Product/2
  Product/1 -> Update NVM RAM/5
  Constant9/1 -> Data Store Write8/1
  Constant10/1 -> Data Store Write10/1
  FloatToFixd_s16_f32/1 -> Update NVM RAM/3
  Constant7/1 -> Update NVM RAM/4

== system SF051A_SnsrOffsLrng/SnsrOffsLrng/SnsrOffsLrngPer1/Learning/ForgettingFactor/Subsystem5 ==

== system SF051A_SnsrOffsLrng/SnsrOffsLrng/SnsrOffsLrngPer1/Learning/HwPos vs HwTrq Model/Subsystem5 ==

== system SF051A_SnsrOffsLrng/SnsrOffsLrng/SnsrOffsLrngPer1/Learning/Recursive Least Square Regression/Calculate Covariance Matrix ==
  note: 'SnsrOffsLrngHwTqLrngTiWghtCoeff' removed from here
  note: (X^T)*(X)
  note: X_k
  note: Mathworks
      | Reference
      | Frame
  note: 3x3
  note: 1x3
  note: 3x1
  note: 3x3
  note: 3x3
  note: 3x3
  note: 3x3
  note: CovMat_k = (I - KVect*XArry)*((CovMat_kPrev)/FF)
      |
      | Where:
      | I = Identity Matrix
      | CovMat_kPrev = Covariance Matrix result the previous iteration.
      | FF = Forgetting Factor (TiWghtCoeff, Time Weight Coefficient)
  XAry : Inport
  KVect : Inport  Port=2
  Data Store Read : DataStoreRead  DataStoreName=SnsrOffsLrnd  DataStoreElements=SnsrOffsLrnd.HwTqLrngCovariMtrx(:,:)
  Data Store Write : DataStoreWrite  RequirementInfo="{'linktype_rmi_doors' '0000babd (/E-STEER Core/SubSystem Specifications/Application Functions/SF051A Sensor Offset Learning)' '#SF051A_174' 'true' 'REQ: SF051A_174' '' ; 'linktype_rmi_doors' '0000babd (/E-STEER Core/SubSystem Specifications/Application Functions/SF051A Sensor Offset Learning)' '#SF051A_173' 'true' 'REQ:  SF051A_173' '' } %GIDa_53e9f122_ab02_4cc9_a40c_de49ec817421"  DataStoreName=SnsrOffsLrnd  DataStoreElements=SnsrOffsLrnd.HwTqLrngCovariMtrx(:,:)
  Identity Matrix : Constant  Value=IDYMTRX_ULS_F32  VectorParams1D=off  OutDataTypeStr=single
  Product : Product  Multiplication=Matrix(*)
  Product1 : Product  Multiplication=Matrix(*)
  Subsystem5 : Subsystem  Description=|  mask(Copyright Information){none=on}
      | Copyright info block.                                               
      |                                                                     
      | Place copyright information at the top of every subsystem in design.
      mask prompts: none "No parameters"
      mask help: Place copyright information at the top of every subsystem in design.
      mask Display:
      | NxtrConf = 'Nexteer Confidential';
      | 
      | sys = bdroot; %handle for the current model ("system")
      | first = get_param(sys,'Created');
      | first = first(end-3:end);  %year is last four digits
      | 
      | last = get_param(sys,'LastModifiedDate');
      | if isempty(last)
      |     last = datestr(now,'yyyy');
      | else
      |     last = last(end-3:end);
      | end
      | 
      | if strcmp(first,last)
      |     fprintf('%s -- Copyright %s Nexteer',NxtrConf,first)
      | else
      |     fprintf('%s -- %s%s- %s Nexteer',NxtrConf,char(169),first,last)
      | end
  Subtract : Sum  Inputs=+-
  wires:
  Product1/1 -> Subtract/2
  KVect/1 -> Product1/1
  XAry/1 -> Product1/2
  Identity Matrix/1 -> Subtract/1
  Subtract/1 -> Product/1
  Product/1 -> Data Store Write/1
  Data Store Read/1 -> Product/2

== system SF051A_SnsrOffsLrng/SnsrOffsLrng/SnsrOffsLrngPer1/Learning/Recursive Least Square Regression/Calculate K Vector ==
  note: Named it KVect instead of KAry because
      | KAry and XAry would look too much alike.
      | Also, XAry  is [1,3]
      |          KVect is [3,1]
  note: (Q+FF)^(-1) scalar
  note: P_kPrev [3x3]
  note: KVect = Q_Temp*(Q+FF)^(-1)
      |
      | Where:
      | Q = (XAry) * (Q_Temp)
      | Q_Temp = (CovMat_kPrev) * (XAry^T)
      | CovMat_kPrev = Covariance Matrix result the previous iteration.
      | FF = Forgetting Factor (TiWghtCoeff, Time Weight Coefficient)
  note: scalar
  note: scalar
  note: X_k [1x3]
  note: X_k [1x3]
  note: X_k [3x1]
  note: Q_Temp [3x1]
  note: Q_Temp [3x1]
  note: K_k [3x1]
  XAry : Inport
  Add2 : Sum
  Data Store Read : DataStoreRead  DataStoreName=SnsrOffsLrnd  DataStoreElements=SnsrOffsLrnd.HwTqLrngCovariMtrx(:,:)
  Divide1 : Product  Inputs=*/
  Forgetting Factor : Constant  RequirementInfo={'linktype_rmi_doors' '0000babd (/E-STEER Core/SubSystem Specifications/Application Functions/SF051A Sensor Offset Learning)' '#SF051A_243' 'true' 'REQ: SF051A_243' '' } %GIDa_0480e113_9aa1_4197_9eb0_4d84996335bf  Value=SnsrOffsLrngHwTqLrngTiWghtCoeff  OutDataTypeStr=single
  Product : Product  Multiplication=Matrix(*)
  Product1 : Product  Multiplication=Matrix(*)
  Subsystem5 : Subsystem  Description=|  mask(Copyright Information){none=on}
      | Copyright info block.                                               
      |                                                                     
      | Place copyright information at the top of every subsystem in design.
      mask prompts: none "No parameters"
      mask help: Place copyright information at the top of every subsystem in design.
      mask Display:
      | NxtrConf = 'Nexteer Confidential';
      | 
      | sys = bdroot; %handle for the current model ("system")
      | first = get_param(sys,'Created');
      | first = first(end-3:end);  %year is last four digits
      | 
      | last = get_param(sys,'LastModifiedDate');
      | if isempty(last)
      |     last = datestr(now,'yyyy');
      | else
      |     last = last(end-3:end);
      | end
      | 
      | if strcmp(first,last)
      |     fprintf('%s -- Copyright %s Nexteer',NxtrConf,first)
      | else
      |     fprintf('%s -- %s%s- %s Nexteer',NxtrConf,char(169),first,last)
      | end
  Transpose : PermuteDimensions
  KVect : Outport
  wires:
  XAry/1 -> Transpose/1, Product1/1
  Data Store Read/1 -> Product/1
  Transpose/1 -> Product/2
  Product/1 -> Product1/2, [Q_Temp]  "QTemp"
  Product1/1 -> Add2/1  "Q"
  Add2/1 -> Divide1/2
  [Q_Temp] -> Divide1/1
  Divide1/1 -> KVect/1  "KVect"
  Forgetting Factor/1 -> Add2/2

== system SF051A_SnsrOffsLrng/SnsrOffsLrng/SnsrOffsLrngPer1/Learning/Recursive Least Square Regression/Subsystem5 ==

== system SF051A_SnsrOffsLrng/SnsrOffsLrng/SnsrOffsLrngPer1/Learning/Recursive Least Square Regression/Update beta_k ==
  note: beta values
  note: Y_k
  note: EstimnVect_k = (EstimnVect_kPrev) + KVect*(HwTqMeasd - XAry *(EstimnVect_kPrev))
      |
      | Where:
      | EstimnVect_k is a vector 3x1 which contains the three estimation [beta_0 ; beta_A1 ; beta_A2 ]
      | EstimnVect_kPrev is the estimations vector of the previous iteration.
  note: 1x3
  note: scalar
  note: 3x1
  note: 3x1
  note: scalar
  note: scalar
  note: 3x1
  note: 3x1
  XAry : Inport
  KVect : Inport  Port=2
  HwTqMeasd : Inport  Port=3
  A1 : Terminator
  Add1 : Sum
  Data Store Read : DataStoreRead  DataStoreName=SnsrOffsLrnd  DataStoreElements=SnsrOffsLrnd.HwTqLrngEstimnVect(:,:)
  Data Store Write : DataStoreWrite  RequirementInfo="{'linktype_rmi_doors' '0000babd (/E-STEER Core/SubSystem Specifications/Application Functions/SF051A Sensor Offset Learning)' '#SF051A_174' 'true' 'REQ:  SF051A_174' '' ; 'linktype_rmi_doors' '0000babd (/E-STEER Core/SubSystem Specifications/Application Functions/SF051A Sensor Offset Learning)' '#SF051A_173' 'true' 'REQ:  SF051A_173' '' } %GIDa_faa57a36_d43e_46b2_93a9_e052c062ee88"  DataStoreName=SnsrOffsLrnd  DataStoreElements=SnsrOffsLrnd.HwTqLrngEstimnVect(:,:)
  Demux : Demux  Outputs=3
  Product : Product  Multiplication=Matrix(*)
  Product1 : Product  Multiplication=Matrix(*)
  Subsystem5 : Subsystem  Description=|  mask(Copyright Information){none=on}
      | Copyright info block.                                               
      |                                                                     
      | Place copyright information at the top of every subsystem in design.
      mask prompts: none "No parameters"
      mask help: Place copyright information at the top of every subsystem in design.
      mask Display:
      | NxtrConf = 'Nexteer Confidential';
      | 
      | sys = bdroot; %handle for the current model ("system")
      | first = get_param(sys,'Created');
      | first = first(end-3:end);  %year is last four digits
      | 
      | last = get_param(sys,'LastModifiedDate');
      | if isempty(last)
      |     last = datestr(now,'yyyy');
      | else
      |     last = last(end-3:end);
      | end
      | 
      | if strcmp(first,last)
      |     fprintf('%s -- Copyright %s Nexteer',NxtrConf,first)
      | else
      |     fprintf('%s -- %s%s- %s Nexteer',NxtrConf,char(169),first,last)
      | end
  Subtract : Sum  Inputs=+-
  HwTqOffsEstimd : Outport
  A2 : Outport  Port=2
  wires:
  XAry/1 -> Product/1
  KVect/1 -> Product1/1
  Product1/1 -> Add1/1
  HwTqMeasd/1 -> Subtract/1
  Product/1 -> Subtract/2
  Subtract/1 -> Product1/2
  Add1/1 -> Data Store Write/1, Demux/1
  Demux/1 -> HwTqOffsEstimd/1  "HwTqOffsEstimd"
  Demux/2 -> A1/1  "A1Estimd"
  Demux/3 -> A2/1  "A2Estimd"
  Data Store Read/1 -> Add1/2, Product/2

== system SF051A_SnsrOffsLrng/SnsrOffsLrng/SnsrOffsLrngPer1/Learning/Update_NvmRam/Subsystem5 ==
